simulink model "AsyncMotor"  (R2025b)
settings: Solver=FixedStepAuto  StartTime=0.0  StopTime=100.0  FixedStep=Ts  RelTol=1e-3
values from neighbouring files (symbols this model uses):
  a_const = 1.0    (= 1)    [constants.m]
  ad_fun_acceleration = 5    [constants.m]
  ad_fun_deceleration = 5    [constants.m]
  fan_abs_delta = abs(fan_max_factor - fan_min_factor)    [constants.m]
  fan_max_factor = 1    [constants.m]
  fan_min_factor = 0.4    [constants.m]
  k_loss = 0.025    [constants.m]
  k_loss0 = 800.0    (= 800)    [constants.m]
  k_rad_AD = 150.0    (= 150)    [constants.m]
  M_AD_nom = 3500.0    (= 3500)    [constants.m]
  M_max_factor = 2.2    [constants.m]
  poles = 2    [constants.m]
  s_max = 0.05    [constants.m]
  T_amb = 25.0    (= 25)    [constants.m]
  tau_AD_base = 900.0    (= 900)    [constants.m]
  Ts = 0.001    [constants.m]
settings Model: TunableVars=P_oil_max,P_oil_min,T_AD_max,T_ballast_max,T_cool_max,omega_ICE_max_prir,omega_ICE_max_run  TunableVarsStorageClass=Auto,Auto,Auto,Auto,Auto,Auto,Auto  TunableVarsTypeQualifier=,,,,,,  Creator=user  LastModifiedBy=user
settings OptimizationCC: DefaultParameterBehavior=Inlined  UseDivisionForNetSlopeComputation=on  GainParamInheritBuiltInType=on  UseFloatMulNetSlope=on  StrengthReduction=on  PassReuseOutputArgsAs=Individual arguments  NoFixptDivByZeroProtection=on  EfficientFloat2IntCast=on  OptimizeBlockOrder=speed  OptimizationPriority=Speed  MultiThreadedLoops=on  AutoScheduleForLoops=on  EfficientTunableParamExpr=on
settings DebuggingCC: ParameterTunabilityLossMsg=error
settings HardwareCC: ProdBitPerLong=64.0  ProdLongLongMode=on  ProdHWDeviceType=Intel->x86-64 (Linux 64)
settings SFSimCC: MATLABDynamicMemAlloc=off  SimTargetLang=C++  SimDLTargetLibrary=mkl-dnn
settings RTWCC: SystemTargetFile=ert.tlc  GenCodeOnly=on  TemplateMakefile=ert_default_tmf  GenerateReport=on  BuildConfiguration=Faster Runs  LaunchReport=on  TargetLang=C++  Description=Embedded Coder
settings CodeAppCC: ForceParamTrailComments=on  IgnoreCustomStorageClasses=off  OperatorAnnotations=on  SimulinkDataObjDesc=on  SFDataObjDesc=on  CustomSymbolStrGlobalVar=rt$N$M  CustomSymbolStrType=$N$M  CustomSymbolStrFcn=$N$M$F  CustomSymbolStrMacro=$N$M  InsertBlockDesc=on
settings ERTTargetCC: InlinedParameterPlacement=Hierarchical  RootIOFormat=Structure reference  ERTCustomFileTemplate=example_file_process.tlc  TargetLangStandard=C++17 (ISO)  GenerateSampleERTMain=on  CodeInterfacePackaging=Reusable function  SupportContinuousTime=on

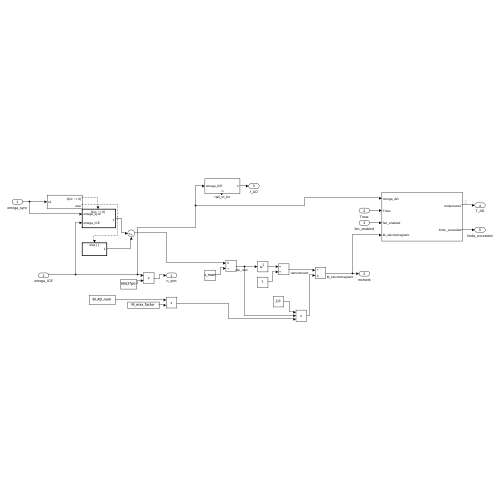
[thumbnail: Simulink's stored preview of the top-level diagram]
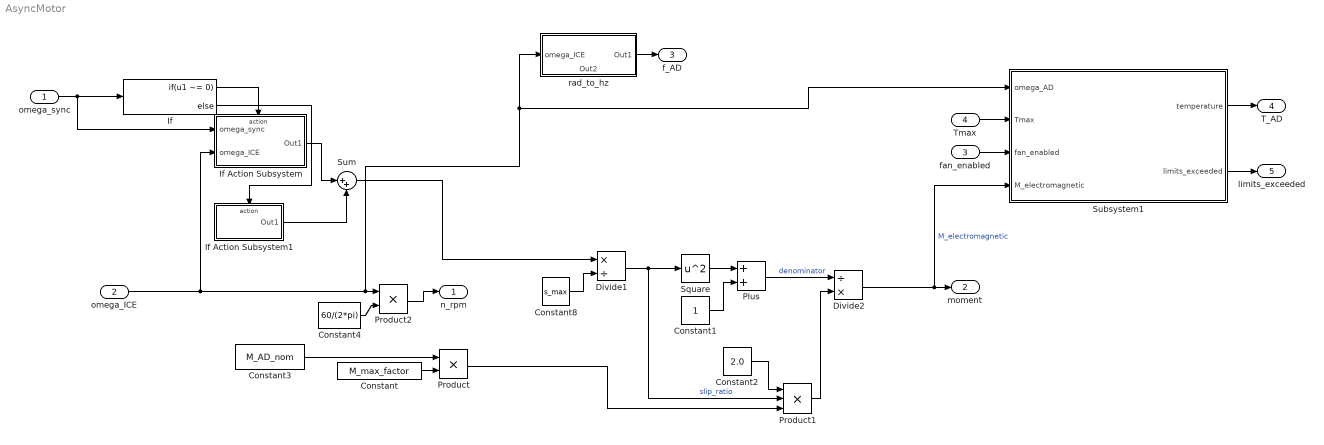
== system AsyncMotor ==
  omega_sync : Inport
  omega_ICE : Inport  Port=2
  fan_enabled : Inport  Port=3
  Tmax : Inport  Port=4
  Constant : Constant  Value=M_max_factor
  Constant1 : Constant
  Constant2 : Constant  Value=2.0
  Constant3 : Constant  Value=M_AD_nom
  Constant4 : Constant  Value=60/(2*pi)
  Constant8 : Constant  Value=s_max
  Divide1 : Product  Inputs=*/
  Divide2 : Product  Inputs=/*
  If : If  IfExpression=u1 ~= 0
  If Action Subsystem : Subsystem  TreatAsAtomicUnit=on
  If Action Subsystem1 : Subsystem  TreatAsAtomicUnit=on
  Plus : Sum
  Product : Product
  Product1 : Product  Inputs=3
  Product2 : Product
  Square : Math  Operator=square
  Subsystem1 : Subsystem
  Sum : Sum  Inputs=|++
  rad_to_hz : Subsystem
      settings: PortSchema="{\"entries\":[{\"content\":{\"sides\":[{\"content\":{\"connectorIds\":[\"In1\"]},\"type\":\"ConnectorPlacement.EquallySpacedRectSide\",\"uuid\":\"cc3fc832-70ea-4290-a79d-d6f32b03a4ae\"},{\"content\":{\"connectorIds\":[\"Out1\"],\"side\":\"RIGHT\"},\"type\":\"ConnectorPlacement.EquallySpacedRectSide\",\"uuid\":\"4026a55a-b470-4e27-a798-f08263e7ed45\"},{\"content\":{\"side\":\"TOP\"},\"type\":\"ConnectorPlacement.EquallySpacedRectSide\",\"uuid\":\"89c8cc72-fd52-4098-bd49-86c4b918072e\"},{\"content\":{\"connectorIds\":[\"Out2\"],\"side\":\"BOTTOM\"},\"type\":\"ConnectorPlacement.EquallySpacedRectSide\",\"uuid\":\"5e9ab07a-d6e4-4a32-a86e-325800baeb71\"}]},\"type\":\"ConnectorPlacement.EquallySpacedConnector\",\"uuid\":\"839d108d-36ac-4b0a-8fe6-036580cd4728\"}],\"packageUris\":[\"http://schema.mathworks.com/mf0/Connector/R2020b\"],\"version\":\"1.0\"}"
  n_rpm : Outport
  moment : Outport  Port=2
  f_AD : Outport  Port=3
  T_AD : Outport  Port=4
  limits_exceeded : Outport  Port=5
  wires:
  omega_sync/1 -> If/1, If Action Subsystem/1(omega_sync)
  Constant8/1 -> Divide1/2
  Divide1/1 -> Product1/2, Square/1  "slip_ratio"
  Product1/1 -> Divide2/2
  Product/1 -> Product1/3
  Constant1/1 -> Plus/2
  Constant/1 -> Product/2
  rad_to_hz/1(Out1) -> f_AD/1
  Plus/1 -> Divide2/1  "denominator"
  Square/1 -> Plus/1
  Constant3/1 -> Product/1
  Divide2/1 -> Subsystem1/4(M_electromagnetic), moment/1  "M_electromagnetic"
  Constant2/1 -> Product1/1
  If/1 -> If Action Subsystem/Action
  If/2 -> If Action Subsystem1/Action
  If Action Subsystem/1(Out1) -> Sum/1
  If Action Subsystem1/1(Out1) -> Sum/2
  Sum/1 -> Divide1/1
  omega_ICE/1 -> If Action Subsystem/2(omega_ICE), Product2/1, Subsystem1/1(omega_AD), rad_to_hz/1(omega_ICE)
  Tmax/1 -> Subsystem1/2(Tmax)
  Subsystem1/1(temperature) -> T_AD/1
  Subsystem1/2(limits_exceeded) -> limits_exceeded/1
  fan_enabled/1 -> Subsystem1/3(fan_enabled)
  Product2/1 -> n_rpm/1
  Constant4/1 -> Product2/2

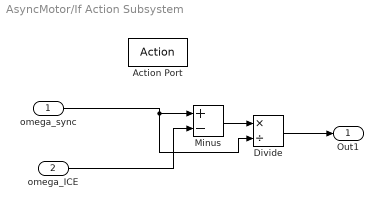
== system AsyncMotor/If Action Subsystem ==
  omega_sync : Inport
  omega_ICE : Inport  Port=2
  Action Port : ActionPort  ActionPortLabel=if(u1 ~= 0)
  Divide : Product  Inputs=*/
  Minus : Sum  Inputs=+-
  Out1 : Outport
  wires:
  Minus/1 -> Divide/1
  omega_ICE/1 -> Minus/2
  omega_sync/1 -> Divide/2, Minus/1
  Divide/1 -> Out1/1

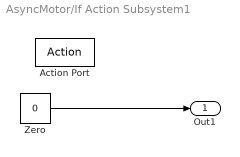
== system AsyncMotor/If Action Subsystem1 ==
  Action Port : ActionPort  ActionPortLabel=else
  Zero : Constant  Value=0  OutDataTypeStr=Inherit: Inherit via back propagation
  Out1 : Outport
  wires:
  Zero/1 -> Out1/1

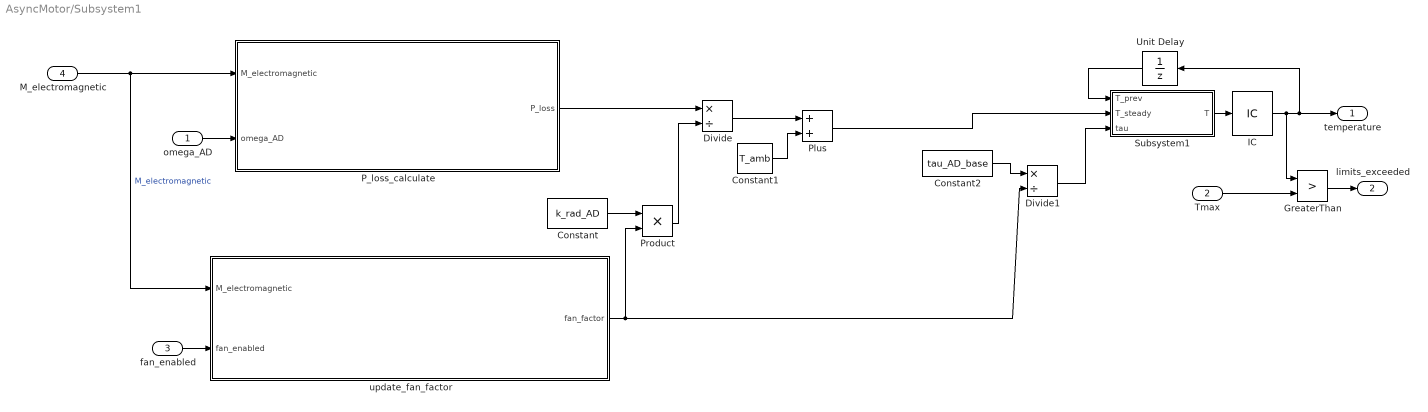
== system AsyncMotor/Subsystem1 ==
  omega_AD : Inport
  Tmax : Inport  Port=2
  fan_enabled : Inport  Port=3
  M_electromagnetic : Inport  Port=4
  Constant : Constant  Value=k_rad_AD
  Constant1 : Constant  Value=T_amb
  Constant2 : Constant  Value=tau_AD_base
  Divide : Product  Inputs=*/
  Divide1 : Product  Inputs=*/
  GreaterThan : RelationalOperator  Operator=>  OutDataTypeStr=boolean  RndMeth=Simplest  InputSameDT=off
  IC : InitialCondition  Value=T_amb
  P_loss_calculate : Subsystem
  Plus : Sum
  Product : Product
  Subsystem1 : Subsystem
  Unit Delay : UnitDelay  InitialCondition=T_amb  SampleTime=-1  HasFrameUpgradeWarning=on
  update_fan_factor : Subsystem
  temperature : Outport
  limits_exceeded : Outport  Port=2
  wires:
  Tmax/1 -> GreaterThan/2
  M_electromagnetic/1 -> update_fan_factor/1(M_electromagnetic), P_loss_calculate/1(M_electromagnetic)  "M_electromagnetic"
  GreaterThan/1 -> limits_exceeded/1
  fan_enabled/1 -> update_fan_factor/2(fan_enabled)
  omega_AD/1 -> P_loss_calculate/2(omega_AD)
  Unit Delay/1 -> Subsystem1/1(T_prev)
  Subsystem1/1(T) -> IC/1
  IC/1 -> GreaterThan/1, Unit Delay/1, temperature/1
  P_loss_calculate/1(P_loss) -> Divide/1
  Constant/1 -> Product/1
  update_fan_factor/1(fan_factor) -> Product/2, Divide1/2
  Product/1 -> Divide/2
  Divide/1 -> Plus/1
  Constant1/1 -> Plus/2
  Plus/1 -> Subsystem1/2(T_steady)
  Divide1/1 -> Subsystem1/3(tau)
  Constant2/1 -> Divide1/1

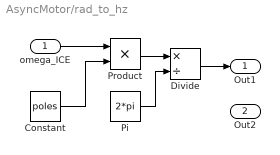
== system AsyncMotor/rad_to_hz ==
  omega_ICE : Inport
  Constant : Constant  Value=poles
  Divide : Product  Inputs=*/
  Pi : Constant  Value=2*pi  OutDataTypeStr=Inherit: Inherit via back propagation
  Product : Product
  Out1 : Outport
  Out2 : Outport  Port=2
  wires:
  Constant/1 -> Product/2
  omega_ICE/1 -> Product/1
  Product/1 -> Divide/1
  Pi/1 -> Divide/2
  Divide/1 -> Out1/1

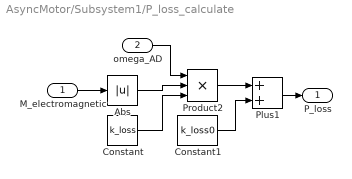
== system AsyncMotor/Subsystem1/P_loss_calculate ==
  M_electromagnetic : Inport
  omega_AD : Inport  Port=2
  Abs : Abs  SaturateOnIntegerOverflow=off
  Constant : Constant  Value=k_loss
  Constant1 : Constant  Value=k_loss0
  Plus1 : Sum
  Product2 : Product  Inputs=3
  P_loss : Outport
  wires:
  Constant/1 -> Product2/3
  M_electromagnetic/1 -> Abs/1
  Product2/1 -> Plus1/1
  omega_AD/1 -> Product2/1
  Constant1/1 -> Plus1/2
  Abs/1 -> Product2/2
  Plus1/1 -> P_loss/1

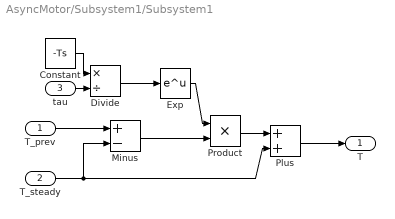
== system AsyncMotor/Subsystem1/Subsystem1 ==
  T_prev : Inport
  T_steady : Inport  Port=2
  tau : Inport  Port=3
  Constant : Constant  Value=-Ts
  Divide : Product  Inputs=*/
  Exp : Math
  Minus : Sum  Inputs=+-
  Plus : Sum
  Product : Product
  T : Outport
  wires:
  T_prev/1 -> Minus/1
  T_steady/1 -> Plus/2, Minus/2
  Minus/1 -> Product/2
  Exp/1 -> Product/1
  Product/1 -> Plus/1
  Plus/1 -> T/1
  tau/1 -> Divide/2
  Constant/1 -> Divide/1
  Divide/1 -> Exp/1

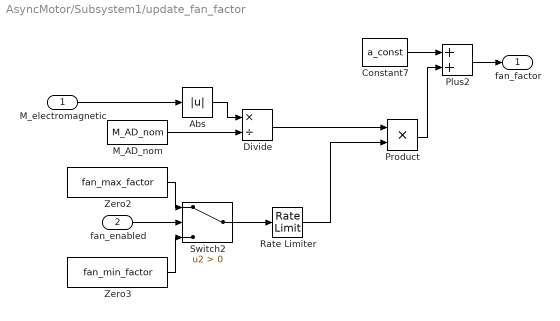
== system AsyncMotor/Subsystem1/update_fan_factor ==
  M_electromagnetic : Inport
  fan_enabled : Inport  Port=2
  Abs : Abs  SaturateOnIntegerOverflow=off
  Constant7 : Constant  Value=a_const
  Divide : Product  Inputs=*/
  M_AD_nom : Constant  Value=M_AD_nom
  Plus2 : Sum
  Product : Product
  Rate Limiter : RateLimiter  RisingSlewLimit=fan_abs_delta/ad_fun_acceleration  FallingSlewLimit=-fan_abs_delta/ad_fun_deceleration
  Switch2 : Switch  Criteria=u2 > Threshold  SaturateOnIntegerOverflow=off  InputSameDT=off
  Zero2 : Constant  Value=fan_max_factor  OutDataTypeStr=Inherit: Inherit via back propagation
  Zero3 : Constant  Value=fan_min_factor  OutDataTypeStr=Inherit: Inherit via back propagation
  fan_factor : Outport
  wires:
  Constant7/1 -> Plus2/1
  Plus2/1 -> fan_factor/1
  M_electromagnetic/1 -> Abs/1
  Abs/1 -> Divide/1
  Zero3/1 -> Switch2/3
  Zero2/1 -> Switch2/1
  fan_enabled/1 -> Switch2/2
  Divide/1 -> Product/1
  Product/1 -> Plus2/2
  M_AD_nom/1 -> Divide/2
  Switch2/1 -> Rate Limiter/1
  Rate Limiter/1 -> Product/2
